simulink model "Height_pid_control"  (R2014a)
settings: Solver=ode45  StartTime=0.0  StopTime=15  RelTol=1e-3
libraries: simulink x1
settings Model: Creator=Felix  LastModifiedBy=Felix

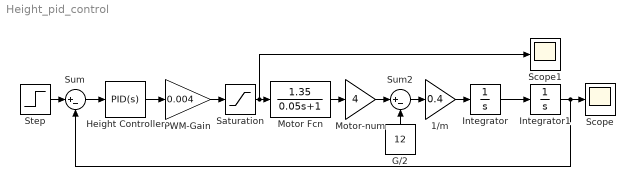
== system Height_pid_control ==
  1/m : Gain  Gain=0.4
  G/2 : Constant  Value=12
  Height Controller : simulink/Continuous/PID Controller  Controller=PID  TimeDomain=Continuous-time  SampleTime=1  IntegratorMethod=Forward Euler  FilterMethod=Forward Euler  Form=Parallel  P=1000  I=700  D=1000  N=100  InitialConditionSource=internal  InitialConditionForIntegrator=0  InitialConditionForFilter=0  ExternalReset=none  LimitOutput=off  UpperSaturationLimit=inf  LowerSaturationLimit=-inf  LinearizeAsGain=on  AntiWindupMode=none  Kb=1  TrackingMode=off  Kt=1  PParamMin=[]  PParamMax=[]  IParamMin=[]  IParamMax=[]  DParamMin=[]  DParamMax=[]  NParamMin=[]  NParamMax=[]  KbParamMin=[]  KbParamMax=[]  KtParamMin=[]  KtParamMax=[]  POutMin=[]  POutMax=[]  IOutMin=[]  IOutMax=[]  DOutMin=[]  DOutMax=[]  NOutMin=[]  NOutMax=[]  KbOutMin=[]  KbOutMax=[]  KtOutMin=[]  KtOutMax=[]  IntegratorOutMin=[]  IntegratorOutMax=[]  FilterOutMin=[]  FilterOutMax=[]  SumOutMin=[]  SumOutMax=[]  SumI1OutMin=[]  SumI1OutMax=[]  SumI2OutMin=[]  SumI2OutMax=[]  SumI3OutMin=[]  SumI3OutMax=[]  SumDOutMin=[]  SumDOutMax=[]  SaturationOutMin=[]  SaturationOutMax=[]  IntegratorContinuousStateAttributes=''  IntegratorStateMustResolveToSignalObject=off  IntegratorRTWStateStorageClass=Auto  FilterContinuousStateAttributes=''  FilterStateMustResolveToSignalObject=off  FilterRTWStateStorageClass=Auto
  Integrator : Integrator
  Integrator1 : Integrator
  Motor Fcn : TransferFcn  Numerator=[1.35]  Denominator=[0.05 1]
  Motor-num : Gain  Gain=4
  PWM-Gain : Gain  Gain=0.004
  Saturation : Saturate  UpperLimit=12  LowerLimit=0
  Scope : Scope
      settings: TimeRange=8.389830508474578  YMin=-0.06858156028368795  YMax=0.08000000000000002
  Scope1 : Scope
  Step : Step  Time=0  SampleTime=0.2
  Sum : Sum  Inputs=|+-
  Sum2 : Sum  Inputs=|+-
  wires:
  Motor Fcn/1 -> Motor-num/1
  Integrator/1 -> Integrator1/1
  Integrator1/1 -> Sum/2, Scope/1
  1/m/1 -> Integrator/1
  Height Controller/1 -> PWM-Gain/1
  Step/1 -> Sum/1
  Sum/1 -> Height Controller/1
  G/2/1 -> Sum2/2
  Motor-num/1 -> Sum2/1
  Sum2/1 -> 1/m/1
  Saturation/1 -> Scope1/1, Motor Fcn/1
  PWM-Gain/1 -> Saturation/1
